simulink model "Zad3"  (R2020b)
settings: Solver=FixedStepAuto  StartTime=0.0  StopTime=300  FixedStep=0.1  RelTol=1e-3
undefined symbols (not defined in the file): kr, Td, Ti, Tp
settings Model: Creator=Maciek  LastModifiedBy=Maciek

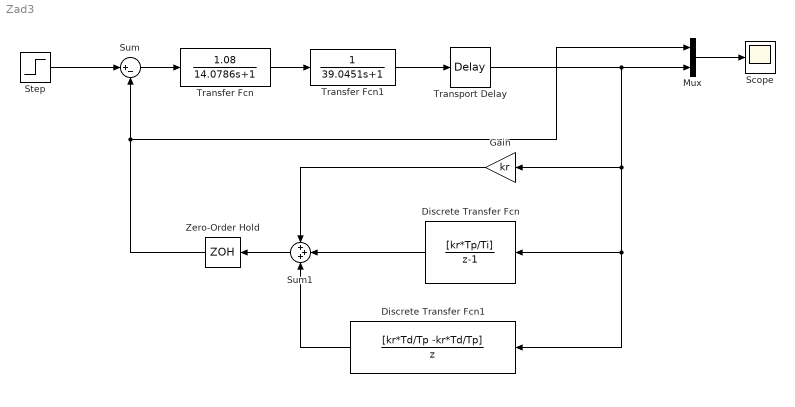
== system Zad3 ==
  Discrete Transfer Fcn : DiscreteTransferFcn  Numerator=[kr*Tp/Ti]  Denominator=[1 -1]
  Discrete Transfer Fcn1 : DiscreteTransferFcn  Numerator=[kr*Td/Tp -kr*Td/Tp]  Denominator=[1 0]
  Gain : Gain  Gain=kr
  Mux : Mux  Inputs=2
  Scope : Scope
  Step : Step  SampleTime=0
  Sum : Sum  Inputs=|+-
  Sum1 : Sum  Inputs=+++
  Transfer Fcn : TransferFcn  Numerator=[1.08]  Denominator=[14.0786 1]
  Transfer Fcn1 : TransferFcn  Denominator=[39.0451 1]
  Transport Delay : TransportDelay  DelayTime=15.1975
  Zero-Order Hold : ZeroOrderHold  SampleTime=Tp
  wires:
  Step/1 -> Sum/1
  Sum/1 -> Transfer Fcn/1
  Transfer Fcn/1 -> Transfer Fcn1/1
  Transfer Fcn1/1 -> Transport Delay/1
  Transport Delay/1 -> Discrete Transfer Fcn1/1, Discrete Transfer Fcn/1, Gain/1, Mux/2
  Gain/1 -> Sum1/1
  Discrete Transfer Fcn/1 -> Sum1/2
  Discrete Transfer Fcn1/1 -> Sum1/3
  Sum1/1 -> Zero-Order Hold/1
  Zero-Order Hold/1 -> Mux/1, Sum/2
  Mux/1 -> Scope/1
